simulink model "Physics_Model"  (R2025b)
settings: Solver=VariableStepAuto  StartTime=0.0  StopTime=10.0  RelTol=1e-3
undefined symbols (not defined in the file or in its folder): config, params
settings Model: Creator=samue  LastModifiedBy=samue

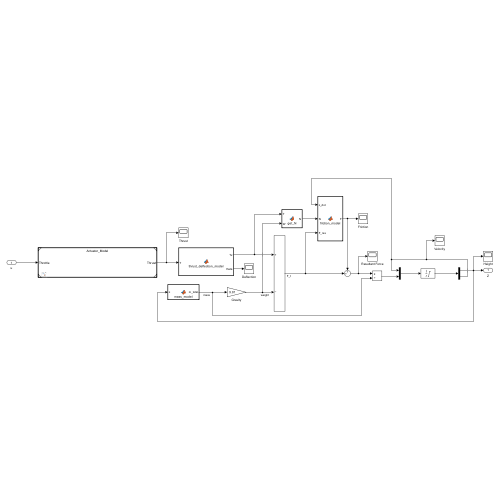
[thumbnail: Simulink's stored preview of the top-level diagram]
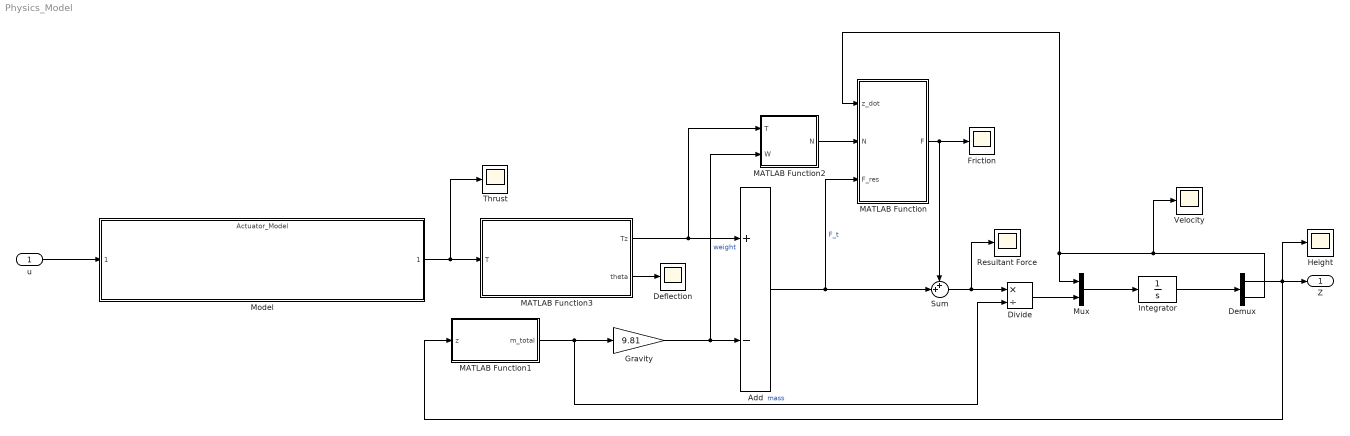
== system Physics_Model ==
  u : Inport
  Add : Sum  Inputs=+-
  Deflection : Scope
  Demux : Demux  Outputs=2
  Divide : Product  Inputs=*/
  Friction : Scope
      settings: DataLoggingVariableName=ScopeData5
  Gravity : Gain  Gain=9.81
  Height : Scope
      settings: DataLoggingVariableName=ScopeData3
  Integrator : Integrator  InitialCondition=[config.initial_height;0]  LimitOutput=on  UpperSaturationLimit=[params.max_height, inf]  LowerSaturationLimit=[params.min_height, -inf]
  MATLAB Function : MATLAB Function  TreatAsAtomicUnit=on
  MATLAB Function1 : MATLAB Function  TreatAsAtomicUnit=on
  MATLAB Function2 : MATLAB Function  TreatAsAtomicUnit=on
  MATLAB Function3 : MATLAB Function  TreatAsAtomicUnit=on
  Model : ModelReference  ModelNameDialog=Actuator_Model.slx  SimulationMode=Normal  ModelReferenceVersion=1.7
  Mux : Mux  Inputs=2
  Resultant Force : Scope
      settings: DataLoggingVariableName=ScopeData4
  Sum : Sum  Inputs=++|
  Thrust : Scope
  Velocity : Scope
      settings: DataLoggingVariableName=ScopeData2
  Z : Outport
  wires:
  Demux/1 -> MATLAB Function1/1(z), Height/1, Z/1
  u/1 -> Model/1
  MATLAB Function1/1(m_total) -> Gravity/1, Divide/2  "mass"
  Gravity/1 -> MATLAB Function2/2(W), Add/2  "weight"
  Add/1 -> MATLAB Function/3(F_res), Sum/2  "F_t"
  Divide/1 -> Mux/2
  Mux/1 -> Integrator/1
  Demux/2 -> Velocity/1, MATLAB Function/1(z_dot), Mux/1
  MATLAB Function/1(F) -> Sum/1, Friction/1
  Sum/1 -> Resultant Force/1, Divide/1
  MATLAB Function2/1(N) -> MATLAB Function/2(N)
  MATLAB Function3/1(Tz) -> MATLAB Function2/1(T), Add/1
  Model/1 -> Thrust/1, MATLAB Function3/1(T)
  MATLAB Function3/2(theta) -> Deflection/1
  Integrator/1 -> Demux/1

== matlab function Physics_Model/MATLAB Function1 ==
  data: z input; m_total output; config parameter
function m_total = mass_model(z, config)
% Calculates total mass of the setup in Kg
    % Extract configuration masses
    m_motor = config.motor_mass;
    m_esc = config.esc_mass;
    m_prop = config.prop_mass;
    m_cable = (config.cable_mass / config.cable_length) * (z - (config.L_cart / 2) + config.cable_length);
    m_frame = 2 * config.arm_mass; 
    m_cart = 0.15;

    % Calculate total mass
    m_total = 2 * (m_motor + m_prop + m_esc) + m_cable + m_frame + m_cart;
end

== matlab function Physics_Model/MATLAB Function ==
  data: F output; z_dot input; N input; F_res input; params parameter
function F = friction_model(z_dot, N, F_res, params)
% Calculates friction force experienced by the track
    v_tol = params.v_tolerance;
    if (abs(z_dot) <= v_tol) && (abs(F_res) < params.Fs_max)
        F = - F_res;
    elseif (abs(z_dot) <= v_tol) && (abs(F_res) >= params.Fs_max)
        F = - sign(F_res) * z_dot;
    else
        F = - sign(z_dot) * N;
    end
end

== matlab function Physics_Model/MATLAB Function2 ==
  data: T input; N output; W input; config parameter
function N = get_N(T, W, config)
% Calculates normal force acting on the cart rail connection
    % Getting moment arms
    L_c = config.cart_length;
    L_cg = config.drone_cg;
    L_m = config.motor_moment_arm_y;
    
    % Taking moment about centre of the cart
    N = (T * L_m - W * L_cg) / L_c;
end

== matlab function Physics_Model/MATLAB Function3 ==
  data: T input; Tz output; theta output
function [Tz, theta] = thrust_deflection_model(T)
% Obtains the structural deflection induced by the thrust and calculates new vertical thrust
    % Get deflection from lookup table (radians)
    theta = 0;

    % Calculate new vertical thrust
    Tz = T * cos(theta);
end
